simulink model "task_5"  (R2023a)
settings: Solver=VariableStepAuto  StartTime=0.0  StopTime=70  RelTol=1e-3  EnableMultiTasking=on
model workspace (MAT data in the model file):
  Tp = 1
  u_liner = 1
settings Model: Creator=Laptop  LastModifiedBy=denys
settings SolverCC: AlgebraicLoopSolver=TrustRegion
settings DataIOCC: ReturnWorkspaceOutputs=off
settings OptimizationCC: LifeSpan=inf
settings DebuggingCC: UnconnectedInputMsg=warning  UnconnectedOutputMsg=warning  UnconnectedLineMsg=warning  SFUnexpectedBacktrackingDiag=warning  SFNoUnconditionalDefaultTransitionDiag=warning  ArithmeticOperatorsInVariantConditions=warning
settings ModelReferenceCC: EnableRefExpFcnMdlSchedulingChecks=on
settings SFSimCC: SimUseLocalCustomCode=off  CustomCodeUndefinedFunction=UseInterfaceOnly
settings RTWCC: RTWUseLocalCustomCode=off
settings CodeAppCC: StateflowObjectComments=on
settings GRTTargetCC: TargetLangStandard=C89/C90 (ANSI)
settings ConfigComp: CovMetricSettings=dw  CovSaveCumulativeToWorkspaceVar=on  CovSaveSingleToWorkspaceVar=on  CovExternalEMLEnable=off

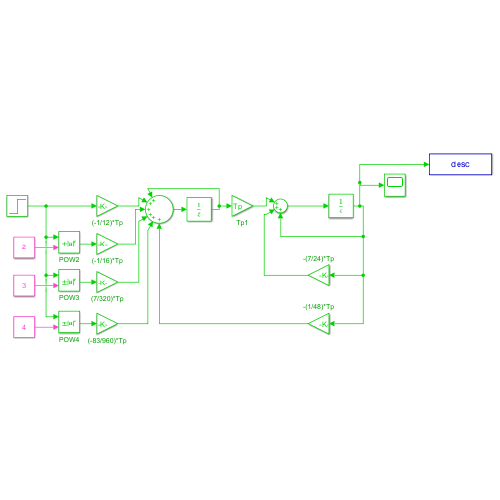
[thumbnail: Simulink's stored preview of the top-level diagram]
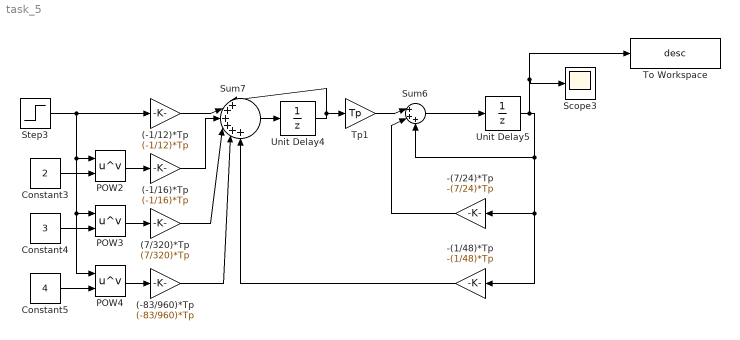
== system task_5 ==
  (-1/12)*Tp : Gain  Gain=(-1/12)*Tp
  (-1/16)*Tp : Gain  Gain=(-1/16)*Tp
  (-83/960)*Tp : Gain  Gain=(-83/960)*Tp
  (7/320)*Tp : Gain  Gain=(7/320)*Tp
  -(1/48)*Tp : Gain  Gain=-(1/48)*Tp
  -(7/24)*Tp : Gain  Gain=-(7/24)*Tp
  Constant3 : Constant  Value=2
  Constant4 : Constant  Value=3
  Constant5 : Constant  Value=4
  POW2 : Math  Operator=pow  SignedPower=on
  POW3 : Math  Operator=pow  SignedPower=on
  POW4 : Math  Operator=pow  SignedPower=on
  Scope3 : Scope
  Step3 : Step  SampleTime=Tp
  Sum6 : Sum  Inputs=|+++
  Sum7 : Sum  Inputs=|++++++
  To Workspace : ToWorkspace  VariableName=desc  SaveFormat=Timeseries  SampleTime=1
  Tp1 : Gain  Gain=Tp
  Unit Delay4 : UnitDelay  SampleTime=Tp  HasFrameUpgradeWarning=on
  Unit Delay5 : UnitDelay  SampleTime=Tp  HasFrameUpgradeWarning=on
  wires:
  Constant3/1 -> POW2/2
  POW4/1 -> (-83/960)*Tp/1
  Unit Delay4/1 -> Sum7/1, Tp1/1
  -(1/48)*Tp/1 -> Sum7/6
  Unit Delay5/1 -> Scope3/1, To Workspace/1, -(1/48)*Tp/1, -(7/24)*Tp/1, Sum6/3
  Constant4/1 -> POW3/2
  Sum7/1 -> Unit Delay4/1
  Step3/1 -> POW4/1, POW3/1, POW2/1, (-1/12)*Tp/1
  Tp1/1 -> Sum6/1
  -(7/24)*Tp/1 -> Sum6/2
  (-1/12)*Tp/1 -> Sum7/2
  Sum6/1 -> Unit Delay5/1
  POW2/1 -> (-1/16)*Tp/1
  POW3/1 -> (7/320)*Tp/1
  (7/320)*Tp/1 -> Sum7/4
  (-1/16)*Tp/1 -> Sum7/3
  Constant5/1 -> POW4/2
  (-83/960)*Tp/1 -> Sum7/5
